simulink model "ddc_bpm_476_066"  (Simulink 7.8)
settings: Solver=ode45  StartTime=0.0  StopTime=2e-3  RelTol=1e-3
undefined symbols (not defined in the file): decim_factor_poly_35, dt_sim, frev_476, Fs_adc, n_ch, n_ovs, R_fofb, R_sec, R_sec_cfir, R_sec_pfir, xlipgetpartsetting
libraries: xbsIndex_r4 x1136, simulink x7
(part 2 of 10)

== system ddc_bpm_476_066/Ksum_tbt_mult2 ==
  In1 : Inport
  In2 : Inport  Port=2
  Cast_truncate1 : Subsystem
  Kx_tbt : xbsIndex_r4/Mult  precision=Full  arith_type="Signed  (2's comp)"  n_bits=16  bin_pt=14  quantization=Truncate  overflow=Wrap  en=off  latency=8  dbl_ovrd=off  use_behavioral_HDL=off  opt=Speed  use_embedded=off  optimum_pipeline=on  pipeline=on  use_rpm=on  placement_style=Triangular  block_type=mult
  Register : xbsIndex_r4/Register  init=0  rst=off  en=off  dbl_ovrd=off  block_type=register
  Out1 : Outport
  wires:
  Kx_tbt/1 -> Cast_truncate1/1(In1)
  In1/1 -> Kx_tbt/1
  Cast_truncate1/1(Out1) -> Register/1
  In2/1 -> Kx_tbt/2
  Register/1 -> Out1/1

== system ddc_bpm_476_066/Ksum_tbt_mult3 ==
  In1 : Inport
  In2 : Inport  Port=2
  Cast_truncate1 : Subsystem
  Kx_tbt : xbsIndex_r4/Mult  precision=Full  arith_type="Signed  (2's comp)"  n_bits=16  bin_pt=14  quantization=Truncate  overflow=Wrap  en=off  latency=8  dbl_ovrd=off  use_behavioral_HDL=off  opt=Speed  use_embedded=off  optimum_pipeline=on  pipeline=on  use_rpm=on  placement_style=Triangular  block_type=mult
  Register : xbsIndex_r4/Register  init=0  rst=off  en=off  dbl_ovrd=off  block_type=register
  Out1 : Outport
  wires:
  Kx_tbt/1 -> Cast_truncate1/1(In1)
  In1/1 -> Kx_tbt/1
  Cast_truncate1/1(Out1) -> Register/1
  In2/1 -> Kx_tbt/2
  Register/1 -> Out1/1

== system ddc_bpm_476_066/Kx_fofb_mult ==
  In1 : Inport
  In2 : Inport  Port=2
  Cast_truncate1 : Subsystem
  Kx_tbt : xbsIndex_r4/Mult  precision=Full  arith_type="Signed  (2's comp)"  n_bits=16  bin_pt=14  quantization=Truncate  overflow=Wrap  en=off  latency=8  dbl_ovrd=off  use_behavioral_HDL=off  opt=Speed  use_embedded=off  optimum_pipeline=on  pipeline=on  use_rpm=on  placement_style=Triangular  block_type=mult
  Register : xbsIndex_r4/Register  init=0  rst=off  en=off  dbl_ovrd=off  block_type=register
  Out1 : Outport
  wires:
  Kx_tbt/1 -> Cast_truncate1/1(In1)
  In1/1 -> Kx_tbt/1
  Cast_truncate1/1(Out1) -> Register/1
  In2/1 -> Kx_tbt/2
  Register/1 -> Out1/1

== system ddc_bpm_476_066/Kx_monit_mult ==
  In1 : Inport
  In2 : Inport  Port=2
  Cast_truncate1 : Subsystem
  Kx_tbt : xbsIndex_r4/Mult  precision=Full  arith_type="Signed  (2's comp)"  n_bits=16  bin_pt=14  quantization=Truncate  overflow=Wrap  en=off  latency=8  dbl_ovrd=off  use_behavioral_HDL=off  opt=Speed  use_embedded=off  optimum_pipeline=on  pipeline=on  use_rpm=on  placement_style=Triangular  block_type=mult
  Register : xbsIndex_r4/Register  init=0  rst=off  en=off  dbl_ovrd=off  block_type=register
  Out1 : Outport
  wires:
  Kx_tbt/1 -> Cast_truncate1/1(In1)
  In1/1 -> Kx_tbt/1
  Cast_truncate1/1(Out1) -> Register/1
  In2/1 -> Kx_tbt/2
  Register/1 -> Out1/1

== system ddc_bpm_476_066/Kx_monit_mult1 ==
  In1 : Inport
  In2 : Inport  Port=2
  Cast_truncate1 : Subsystem
  Kx_tbt : xbsIndex_r4/Mult  precision=Full  arith_type="Signed  (2's comp)"  n_bits=16  bin_pt=14  quantization=Truncate  overflow=Wrap  en=off  latency=8  dbl_ovrd=off  use_behavioral_HDL=off  opt=Speed  use_embedded=off  optimum_pipeline=on  pipeline=on  use_rpm=on  placement_style=Triangular  block_type=mult
  Register : xbsIndex_r4/Register  init=0  rst=off  en=off  dbl_ovrd=off  block_type=register
  Out1 : Outport
  wires:
  Kx_tbt/1 -> Cast_truncate1/1(In1)
  In1/1 -> Kx_tbt/1
  Cast_truncate1/1(Out1) -> Register/1
  In2/1 -> Kx_tbt/2
  Register/1 -> Out1/1

== system ddc_bpm_476_066/Kx_q_fofb_mult ==
  In1 : Inport
  In2 : Inport  Port=2
  Cast_truncate1 : Subsystem
  Kx_tbt : xbsIndex_r4/Mult  precision=Full  arith_type="Signed  (2's comp)"  n_bits=16  bin_pt=14  quantization=Truncate  overflow=Wrap  en=off  latency=8  dbl_ovrd=off  use_behavioral_HDL=off  opt=Speed  use_embedded=off  optimum_pipeline=on  pipeline=on  use_rpm=on  placement_style=Triangular  block_type=mult
  Register : xbsIndex_r4/Register  init=0  rst=off  en=off  dbl_ovrd=off  block_type=register
  Out1 : Outport
  wires:
  Kx_tbt/1 -> Cast_truncate1/1(In1)
  In1/1 -> Kx_tbt/1
  Cast_truncate1/1(Out1) -> Register/1
  In2/1 -> Kx_tbt/2
  Register/1 -> Out1/1

== system ddc_bpm_476_066/Kx_q_fofb_mult1 ==
  In1 : Inport
  In2 : Inport  Port=2
  Cast_truncate1 : Subsystem
  Kx_tbt : xbsIndex_r4/Mult  precision=Full  arith_type="Signed  (2's comp)"  n_bits=16  bin_pt=14  quantization=Truncate  overflow=Wrap  en=off  latency=8  dbl_ovrd=off  use_behavioral_HDL=off  opt=Speed  use_embedded=off  optimum_pipeline=on  pipeline=on  use_rpm=on  placement_style=Triangular  block_type=mult
  Register : xbsIndex_r4/Register  init=0  rst=off  en=off  dbl_ovrd=off  block_type=register
  Out1 : Outport
  wires:
  Kx_tbt/1 -> Cast_truncate1/1(In1)
  In1/1 -> Kx_tbt/1
  Cast_truncate1/1(Out1) -> Register/1
  In2/1 -> Kx_tbt/2
  Register/1 -> Out1/1

== system ddc_bpm_476_066/Kx_q_fofb_mult2 ==
  In1 : Inport
  In2 : Inport  Port=2
  Cast_truncate1 : Subsystem
  Kx_tbt : xbsIndex_r4/Mult  precision=Full  arith_type="Signed  (2's comp)"  n_bits=16  bin_pt=14  quantization=Truncate  overflow=Wrap  en=off  latency=8  dbl_ovrd=off  use_behavioral_HDL=off  opt=Speed  use_embedded=off  optimum_pipeline=on  pipeline=on  use_rpm=on  placement_style=Triangular  block_type=mult
  Register : xbsIndex_r4/Register  init=0  rst=off  en=off  dbl_ovrd=off  block_type=register
  Out1 : Outport
  wires:
  Kx_tbt/1 -> Cast_truncate1/1(In1)
  In1/1 -> Kx_tbt/1
  Cast_truncate1/1(Out1) -> Register/1
  In2/1 -> Kx_tbt/2
  Register/1 -> Out1/1

== system ddc_bpm_476_066/Kx_q_monit_mult ==
  In1 : Inport
  In2 : Inport  Port=2
  Cast_truncate1 : Subsystem
  Kx_tbt : xbsIndex_r4/Mult  precision=Full  arith_type="Signed  (2's comp)"  n_bits=16  bin_pt=14  quantization=Truncate  overflow=Wrap  en=off  latency=8  dbl_ovrd=off  use_behavioral_HDL=off  opt=Speed  use_embedded=off  optimum_pipeline=on  pipeline=on  use_rpm=on  placement_style=Triangular  block_type=mult
  Register : xbsIndex_r4/Register  init=0  rst=off  en=off  dbl_ovrd=off  block_type=register
  Out1 : Outport
  wires:
  Kx_tbt/1 -> Cast_truncate1/1(In1)
  In1/1 -> Kx_tbt/1
  Cast_truncate1/1(Out1) -> Register/1
  In2/1 -> Kx_tbt/2
  Register/1 -> Out1/1

== system ddc_bpm_476_066/Kx_q_monit_mult1 ==
  In1 : Inport
  In2 : Inport  Port=2
  Cast_truncate1 : Subsystem
  Kx_tbt : xbsIndex_r4/Mult  precision=Full  arith_type="Signed  (2's comp)"  n_bits=16  bin_pt=14  quantization=Truncate  overflow=Wrap  en=off  latency=8  dbl_ovrd=off  use_behavioral_HDL=off  opt=Speed  use_embedded=off  optimum_pipeline=on  pipeline=on  use_rpm=on  placement_style=Triangular  block_type=mult
  Register : xbsIndex_r4/Register  init=0  rst=off  en=off  dbl_ovrd=off  block_type=register
  Out1 : Outport
  wires:
  Kx_tbt/1 -> Cast_truncate1/1(In1)
  In1/1 -> Kx_tbt/1
  Cast_truncate1/1(Out1) -> Register/1
  In2/1 -> Kx_tbt/2
  Register/1 -> Out1/1

== system ddc_bpm_476_066/Kx_q_tbt_mult ==
  In1 : Inport
  In2 : Inport  Port=2
  Cast_truncate1 : Subsystem
  Kx_tbt : xbsIndex_r4/Mult  precision=Full  arith_type="Signed  (2's comp)"  n_bits=16  bin_pt=14  quantization=Truncate  overflow=Wrap  en=off  latency=8  dbl_ovrd=off  use_behavioral_HDL=off  opt=Speed  use_embedded=off  optimum_pipeline=on  pipeline=on  use_rpm=on  placement_style=Triangular  block_type=mult
  Register : xbsIndex_r4/Register  init=0  rst=off  en=off  dbl_ovrd=off  block_type=register
  Out1 : Outport
  wires:
  Kx_tbt/1 -> Cast_truncate1/1(In1)
  In1/1 -> Kx_tbt/1
  Cast_truncate1/1(Out1) -> Register/1
  In2/1 -> Kx_tbt/2
  Register/1 -> Out1/1

== system ddc_bpm_476_066/Kx_tbt_mult ==
  In1 : Inport
  In2 : Inport  Port=2
  Cast_truncate1 : Subsystem
  Kx_tbt : xbsIndex_r4/Mult  precision=Full  arith_type="Signed  (2's comp)"  n_bits=16  bin_pt=14  quantization=Truncate  overflow=Wrap  en=off  latency=8  dbl_ovrd=off  use_behavioral_HDL=off  opt=Speed  use_embedded=off  optimum_pipeline=on  pipeline=on  use_rpm=on  placement_style=Triangular  block_type=mult
  Register : xbsIndex_r4/Register  init=0  rst=off  en=off  dbl_ovrd=off  block_type=register
  Out1 : Outport
  wires:
  Kx_tbt/1 -> Cast_truncate1/1(In1)
  In1/1 -> Kx_tbt/1
  Cast_truncate1/1(Out1) -> Register/1
  In2/1 -> Kx_tbt/2
  Register/1 -> Out1/1

== system ddc_bpm_476_066/Ky_tbt_mult ==
  In1 : Inport
  In2 : Inport  Port=2
  Cast_truncate1 : Subsystem
  Ky_tbt : xbsIndex_r4/Mult  precision=Full  arith_type="Signed  (2's comp)"  n_bits=16  bin_pt=14  quantization=Truncate  overflow=Wrap  en=off  latency=8  dbl_ovrd=off  use_behavioral_HDL=off  opt=Speed  use_embedded=off  optimum_pipeline=on  pipeline=on  use_rpm=on  placement_style=Triangular  block_type=mult
  Register : xbsIndex_r4/Register  init=0  rst=off  en=off  dbl_ovrd=off  block_type=register
  Out1 : Outport
  wires:
  Ky_tbt/1 -> Cast_truncate1/1(In1)
  In1/1 -> Ky_tbt/1
  Cast_truncate1/1(Out1) -> Register/1
  In2/1 -> Ky_tbt/2
  Register/1 -> Out1/1

== system ddc_bpm_476_066/Ky_tbt_mult1 ==
  In1 : Inport
  In2 : Inport  Port=2
  Cast_truncate1 : Subsystem
  Kx_tbt : xbsIndex_r4/Mult  precision=Full  arith_type="Signed  (2's comp)"  n_bits=16  bin_pt=14  quantization=Truncate  overflow=Wrap  en=off  latency=8  dbl_ovrd=off  use_behavioral_HDL=off  opt=Speed  use_embedded=off  optimum_pipeline=on  pipeline=on  use_rpm=on  placement_style=Triangular  block_type=mult
  Register : xbsIndex_r4/Register  init=0  rst=off  en=off  dbl_ovrd=off  block_type=register
  Out1 : Outport
  wires:
  Kx_tbt/1 -> Cast_truncate1/1(In1)
  In1/1 -> Kx_tbt/1
  Cast_truncate1/1(Out1) -> Register/1
  In2/1 -> Kx_tbt/2
  Register/1 -> Out1/1

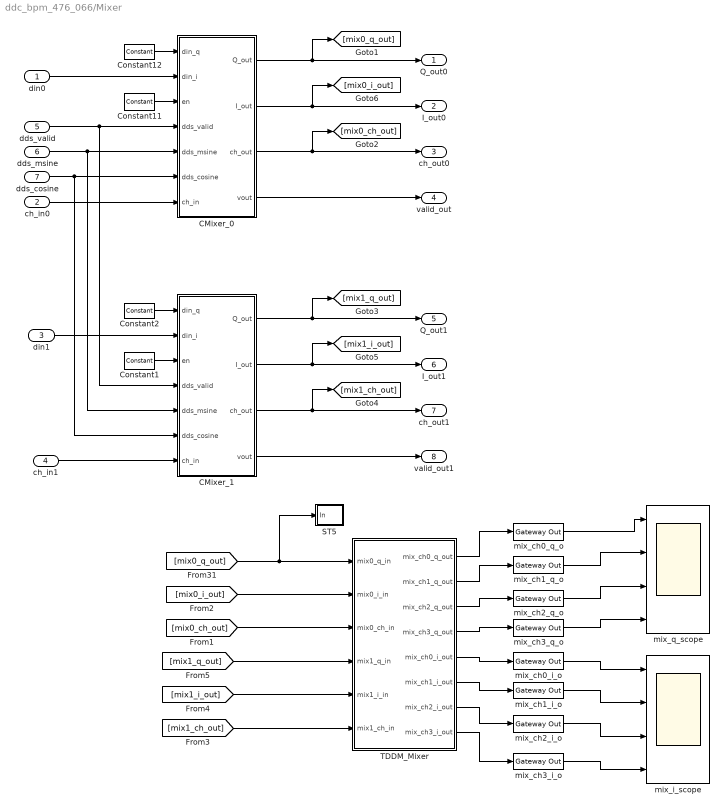
== system ddc_bpm_476_066/Mixer ==
  din0 : Inport
  ch_in0 : Inport  Port=2
  din1 : Inport  Port=3
  ch_in1 : Inport  Port=4
  dds_valid : Inport  Port=5
  dds_msine : Inport  Port=6
  dds_cosine : Inport  Port=7
  CMixer_0 : Subsystem
  CMixer_1 : Subsystem
  Constant1 : xbsIndex_r4/Constant  const=1  gui_display_data_type=Boolean  arith_type=Boolean  n_bits=24  bin_pt=22  preci_type=Single  exp_width=8  frac_width=24  explicit_period=on  period=dt_sim  equ=P=C  opselect=C  inp2=PCIN>>17  opr=+  inp1=P  carry=CIN  dbl_ovrd=off  block_type=constant
  Constant11 : xbsIndex_r4/Constant  const=1  gui_display_data_type=Boolean  arith_type=Boolean  n_bits=24  bin_pt=22  preci_type=Single  exp_width=8  frac_width=24  explicit_period=on  period=dt_sim  equ=P=C  opselect=C  inp2=PCIN>>17  opr=+  inp1=P  carry=CIN  dbl_ovrd=off  block_type=constant
  Constant12 : xbsIndex_r4/Constant  const=0  gui_display_data_type=Fixed-point  arith_type=Signed (2's comp)  n_bits=24  bin_pt=22  preci_type=Single  exp_width=8  frac_width=24  explicit_period=on  period=dt_sim  equ=P=C  opselect=C  inp2=PCIN>>17  opr=+  inp1=P  carry=CIN  dbl_ovrd=off  block_type=constant
  Constant2 : xbsIndex_r4/Constant  const=0  gui_display_data_type=Fixed-point  arith_type=Signed (2's comp)  n_bits=24  bin_pt=22  preci_type=Single  exp_width=8  frac_width=24  explicit_period=on  period=dt_sim  equ=P=C  opselect=C  inp2=PCIN>>17  opr=+  inp1=P  carry=CIN  dbl_ovrd=off  block_type=constant
  ST5 : Subsystem
  TDDM_Mixer : Subsystem
  mix_ch0_i_o : xbsIndex_r4/Gateway Out  inherit_from_input=on  hdl_port=on  timing_constraint=Data Rate  locs_specified=off  LOCs={}  UseAsDAC=off  DACChannel='1'  block_type=gatewayout
      settings: infoedit="Gateway out block.  Converts Xilinx fixed-point or floating-point type inputs into ouputs of type Simulink integer, single, double, or fixed point.<br><br>Hardware notes:  In hardware these blocks become top level output ports or are discarded, depending on how they are configured."
  mix_ch0_q_o : xbsIndex_r4/Gateway Out  inherit_from_input=on  hdl_port=on  timing_constraint=Data Rate  locs_specified=off  LOCs={}  UseAsDAC=off  DACChannel='1'  block_type=gatewayout
      settings: infoedit="Gateway out block.  Converts Xilinx fixed-point or floating-point type inputs into ouputs of type Simulink integer, single, double, or fixed point.<br><br>Hardware notes:  In hardware these blocks become top level output ports or are discarded, depending on how they are configured."
  mix_ch1_i_o : xbsIndex_r4/Gateway Out  inherit_from_input=on  hdl_port=on  timing_constraint=Data Rate  locs_specified=off  LOCs={}  UseAsDAC=off  DACChannel='1'  block_type=gatewayout
      settings: infoedit="Gateway out block.  Converts Xilinx fixed-point or floating-point type inputs into ouputs of type Simulink integer, single, double, or fixed point.<br><br>Hardware notes:  In hardware these blocks become top level output ports or are discarded, depending on how they are configured."
  mix_ch1_q_o : xbsIndex_r4/Gateway Out  inherit_from_input=on  hdl_port=on  timing_constraint=Data Rate  locs_specified=off  LOCs={}  UseAsDAC=off  DACChannel='1'  block_type=gatewayout
      settings: infoedit="Gateway out block.  Converts Xilinx fixed-point or floating-point type inputs into ouputs of type Simulink integer, single, double, or fixed point.<br><br>Hardware notes:  In hardware these blocks become top level output ports or are discarded, depending on how they are configured."
  mix_ch2_i_o : xbsIndex_r4/Gateway Out  inherit_from_input=on  hdl_port=on  timing_constraint=Data Rate  locs_specified=off  LOCs={}  UseAsDAC=off  DACChannel='1'  block_type=gatewayout
      settings: infoedit="Gateway out block.  Converts Xilinx fixed-point or floating-point type inputs into ouputs of type Simulink integer, single, double, or fixed point.<br><br>Hardware notes:  In hardware these blocks become top level output ports or are discarded, depending on how they are configured."
  mix_ch2_q_o : xbsIndex_r4/Gateway Out  inherit_from_input=on  hdl_port=on  timing_constraint=Data Rate  locs_specified=off  LOCs={}  UseAsDAC=off  DACChannel='1'  block_type=gatewayout
      settings: infoedit="Gateway out block.  Converts Xilinx fixed-point or floating-point type inputs into ouputs of type Simulink integer, single, double, or fixed point.<br><br>Hardware notes:  In hardware these blocks become top level output ports or are discarded, depending on how they are configured."
  mix_ch3_i_o : xbsIndex_r4/Gateway Out  inherit_from_input=on  hdl_port=on  timing_constraint=Data Rate  locs_specified=off  LOCs={}  UseAsDAC=off  DACChannel='1'  block_type=gatewayout
      settings: infoedit="Gateway out block.  Converts Xilinx fixed-point or floating-point type inputs into ouputs of type Simulink integer, single, double, or fixed point.<br><br>Hardware notes:  In hardware these blocks become top level output ports or are discarded, depending on how they are configured."
  mix_ch3_q_o : xbsIndex_r4/Gateway Out  inherit_from_input=on  hdl_port=on  timing_constraint=Data Rate  locs_specified=off  LOCs={}  UseAsDAC=off  DACChannel='1'  block_type=gatewayout
      settings: infoedit="Gateway out block.  Converts Xilinx fixed-point or floating-point type inputs into ouputs of type Simulink integer, single, double, or fixed point.<br><br>Hardware notes:  In hardware these blocks become top level output ports or are discarded, depending on how they are configured."
  mix_i_scope : Scope  NumInputPorts=4
      settings: TimeRange=0.00011214  YMin=-0.1~-1.5~-0.002~-1.5  YMax=1~1.5~0.00075~1.5  SaveName=ScopeData14  MaxDataPoints=1000000  SampleInput=on
  mix_q_scope : Scope  NumInputPorts=4
      settings: TimeRange=0.00011214  YMin=-0.1~-1.5~-0.002~-1.5  YMax=1~1.5~0.00075~1.5  SaveName=ScopeData13  MaxDataPoints=1000000  SampleInput=on
  Q_out0 : Outport
  I_out0 : Outport  Port=2
  ch_out0 : Outport  Port=3
  valid_out : Outport  Port=4
  Q_out1 : Outport  Port=5
  I_out1 : Outport  Port=6
  ch_out1 : Outport  Port=7
  valid_out1 : Outport  Port=8
  wires:
  Constant12/1 -> CMixer_0/1(din_q)
  Constant11/1 -> CMixer_0/3(en)
  CMixer_0/1(Q_out) -> Q_out0/1, [mix0_q_out]
  din0/1 -> CMixer_0/2(din_i)
  CMixer_0/2(I_out) -> I_out0/1, [mix0_i_out]
  dds_valid/1 -> CMixer_0/4(dds_valid), CMixer_1/4(dds_valid)
  dds_cosine/1 -> CMixer_0/6(dds_cosine), CMixer_1/6(dds_cosine)
  CMixer_0/3(ch_out) -> ch_out0/1, [mix0_ch_out]
  dds_msine/1 -> CMixer_0/5(dds_msine), CMixer_1/5(dds_msine)
  CMixer_0/4(vout) -> valid_out/1
  ch_in0/1 -> CMixer_0/7(ch_in)
  [mix0_q_out] -> TDDM_Mixer/1(mix0_q_in), ST5/1(In)
  [mix0_ch_out] -> TDDM_Mixer/3(mix0_ch_in)
  [mix0_i_out] -> TDDM_Mixer/2(mix0_i_in)
  TDDM_Mixer/1(mix_ch0_q_out) -> mix_ch0_q_o/1
  TDDM_Mixer/2(mix_ch1_q_out) -> mix_ch1_q_o/1
  TDDM_Mixer/3(mix_ch2_q_out) -> mix_ch2_q_o/1
  TDDM_Mixer/4(mix_ch3_q_out) -> mix_ch3_q_o/1
  TDDM_Mixer/5(mix_ch0_i_out) -> mix_ch0_i_o/1
  TDDM_Mixer/6(mix_ch1_i_out) -> mix_ch1_i_o/1
  TDDM_Mixer/7(mix_ch2_i_out) -> mix_ch2_i_o/1
  TDDM_Mixer/8(mix_ch3_i_out) -> mix_ch3_i_o/1
  mix_ch0_i_o/1 -> mix_i_scope/1
  mix_ch1_i_o/1 -> mix_i_scope/2
  mix_ch2_i_o/1 -> mix_i_scope/3
  mix_ch3_i_o/1 -> mix_i_scope/4
  mix_ch3_q_o/1 -> mix_q_scope/4
  mix_ch2_q_o/1 -> mix_q_scope/3
  mix_ch1_q_o/1 -> mix_q_scope/2
  mix_ch0_q_o/1 -> mix_q_scope/1
  Constant2/1 -> CMixer_1/1(din_q)
  Constant1/1 -> CMixer_1/3(en)
  CMixer_1/1(Q_out) -> Q_out1/1, [mix1_q_out]
  din1/1 -> CMixer_1/2(din_i)
  CMixer_1/2(I_out) -> I_out1/1, [mix1_i_out]
  CMixer_1/3(ch_out) -> ch_out1/1, [mix1_ch_out]
  CMixer_1/4(vout) -> valid_out1/1
  ch_in1/1 -> CMixer_1/7(ch_in)
  [mix1_q_out] -> TDDM_Mixer/4(mix1_q_in)
  [mix1_i_out] -> TDDM_Mixer/5(mix1_i_in)
  [mix1_ch_out] -> TDDM_Mixer/6(mix1_ch_in)

== system ddc_bpm_476_066/Monit_amp ==
  din : Inport
  ch_in : Inport  Port=2
  Monit_amp_c : Subsystem
  TDDM_monit_amp_out : Subsystem
  Terminator5 : Terminator
  amp_out0 : Outport
  amp_out1 : Outport  Port=2
  amp_out2 : Outport  Port=3
  amp_out3 : Outport  Port=4
  wires:
  Monit_amp_c/1(amp_out) -> TDDM_monit_amp_out/1(monit_amp_din)
  Monit_amp_c/2(ch_out) -> TDDM_monit_amp_out/2(monit_amp_ch_in)
  Monit_amp_c/3(valid_out) -> Terminator5/1
  TDDM_monit_amp_out/1(monit_amp_data0_out) -> amp_out0/1
  din/1 -> Monit_amp_c/1(din)
  TDDM_monit_amp_out/2(monit_amp_data1_out) -> amp_out1/1
  TDDM_monit_amp_out/3(monit_amp_data2_out) -> amp_out2/1
  ch_in/1 -> Monit_amp_c/2(ch_in)
  TDDM_monit_amp_out/4(monit_amp_data3_out) -> amp_out3/1

== system ddc_bpm_476_066/ST1 ==
  In : Inport
  Display : Display
  Sample Time : xbsIndex_r4/Sample Time  block_type=sampletime
      settings: infoedit="The Sample Time block reports the normalized sample period of its input.  A signal's normalized sample period is not equivalent to its Simulink absolute sample period.<br><br>Hardware notes: This block is implemented as a constant in hardware."
  out : xbsIndex_r4/Gateway Out  inherit_from_input=on  hdl_port=off  timing_constraint=Data Rate  locs_specified=off  LOCs={}  UseAsDAC=off  DACChannel='1'  block_type=gatewayout
      settings: infoedit="Gateway out block.  Converts Xilinx fixed-point or floating-point type inputs into ouputs of type Simulink integer, single, double, or fixed point.<br><br>Hardware notes:  In hardware these blocks become top level output ports or are discarded, depending on how they are configured."
  wires:
  out/1 -> Display/1
  Sample Time/1 -> out/1
  In/1 -> Sample Time/1

== system ddc_bpm_476_066/ST10 ==
  In : Inport
  Display : Display
  Sample Time : xbsIndex_r4/Sample Time  block_type=sampletime
      settings: infoedit="The Sample Time block reports the normalized sample period of its input.  A signal's normalized sample period is not equivalent to its Simulink absolute sample period.<br><br>Hardware notes: This block is implemented as a constant in hardware."
  out : xbsIndex_r4/Gateway Out  inherit_from_input=on  hdl_port=off  timing_constraint=Data Rate  locs_specified=off  LOCs={}  UseAsDAC=off  DACChannel='1'  block_type=gatewayout
      settings: infoedit="Gateway out block.  Converts Xilinx fixed-point or floating-point type inputs into ouputs of type Simulink integer, single, double, or fixed point.<br><br>Hardware notes:  In hardware these blocks become top level output ports or are discarded, depending on how they are configured."
  wires:
  out/1 -> Display/1
  Sample Time/1 -> out/1
  In/1 -> Sample Time/1

== system ddc_bpm_476_066/ST2 ==
  In : Inport
  Display : Display
  Sample Time : xbsIndex_r4/Sample Time  block_type=sampletime
      settings: infoedit="The Sample Time block reports the normalized sample period of its input.  A signal's normalized sample period is not equivalent to its Simulink absolute sample period.<br><br>Hardware notes: This block is implemented as a constant in hardware."
  out : xbsIndex_r4/Gateway Out  inherit_from_input=on  hdl_port=off  timing_constraint=Data Rate  locs_specified=off  LOCs={}  UseAsDAC=off  DACChannel='1'  block_type=gatewayout
      settings: infoedit="Gateway out block.  Converts Xilinx fixed-point or floating-point type inputs into ouputs of type Simulink integer, single, double, or fixed point.<br><br>Hardware notes:  In hardware these blocks become top level output ports or are discarded, depending on how they are configured."
  wires:
  out/1 -> Display/1
  Sample Time/1 -> out/1
  In/1 -> Sample Time/1

== system ddc_bpm_476_066/ST3 ==
  In : Inport
  Display : Display
  Sample Time : xbsIndex_r4/Sample Time  block_type=sampletime
      settings: infoedit="The Sample Time block reports the normalized sample period of its input.  A signal's normalized sample period is not equivalent to its Simulink absolute sample period.<br><br>Hardware notes: This block is implemented as a constant in hardware."
  out : xbsIndex_r4/Gateway Out  inherit_from_input=on  hdl_port=off  timing_constraint=Data Rate  locs_specified=off  LOCs={}  UseAsDAC=off  DACChannel='1'  block_type=gatewayout
      settings: infoedit="Gateway out block.  Converts Xilinx fixed-point or floating-point type inputs into ouputs of type Simulink integer, single, double, or fixed point.<br><br>Hardware notes:  In hardware these blocks become top level output ports or are discarded, depending on how they are configured."
  wires:
  out/1 -> Display/1
  Sample Time/1 -> out/1
  In/1 -> Sample Time/1

== system ddc_bpm_476_066/ST4 ==
  In : Inport
  Display : Display
  Sample Time : xbsIndex_r4/Sample Time  block_type=sampletime
      settings: infoedit="The Sample Time block reports the normalized sample period of its input.  A signal's normalized sample period is not equivalent to its Simulink absolute sample period.<br><br>Hardware notes: This block is implemented as a constant in hardware."
  out : xbsIndex_r4/Gateway Out  inherit_from_input=on  hdl_port=off  timing_constraint=Data Rate  locs_specified=off  LOCs={}  UseAsDAC=off  DACChannel='1'  block_type=gatewayout
      settings: infoedit="Gateway out block.  Converts Xilinx fixed-point or floating-point type inputs into ouputs of type Simulink integer, single, double, or fixed point.<br><br>Hardware notes:  In hardware these blocks become top level output ports or are discarded, depending on how they are configured."
  wires:
  out/1 -> Display/1
  Sample Time/1 -> out/1
  In/1 -> Sample Time/1

== system ddc_bpm_476_066/ST5 ==
  In : Inport
  Display : Display
  Sample Time : xbsIndex_r4/Sample Time  block_type=sampletime
      settings: infoedit="The Sample Time block reports the normalized sample period of its input.  A signal's normalized sample period is not equivalent to its Simulink absolute sample period.<br><br>Hardware notes: This block is implemented as a constant in hardware."
  out : xbsIndex_r4/Gateway Out  inherit_from_input=on  hdl_port=off  timing_constraint=Data Rate  locs_specified=off  LOCs={}  UseAsDAC=off  DACChannel='1'  block_type=gatewayout
      settings: infoedit="Gateway out block.  Converts Xilinx fixed-point or floating-point type inputs into ouputs of type Simulink integer, single, double, or fixed point.<br><br>Hardware notes:  In hardware these blocks become top level output ports or are discarded, depending on how they are configured."
  wires:
  out/1 -> Display/1
  Sample Time/1 -> out/1
  In/1 -> Sample Time/1

== system ddc_bpm_476_066/ST6 ==
  In : Inport
  Display : Display
  Sample Time : xbsIndex_r4/Sample Time  block_type=sampletime
      settings: infoedit="The Sample Time block reports the normalized sample period of its input.  A signal's normalized sample period is not equivalent to its Simulink absolute sample period.<br><br>Hardware notes: This block is implemented as a constant in hardware."
  out : xbsIndex_r4/Gateway Out  inherit_from_input=on  hdl_port=off  timing_constraint=Data Rate  locs_specified=off  LOCs={}  UseAsDAC=off  DACChannel='1'  block_type=gatewayout
      settings: infoedit="Gateway out block.  Converts Xilinx fixed-point or floating-point type inputs into ouputs of type Simulink integer, single, double, or fixed point.<br><br>Hardware notes:  In hardware these blocks become top level output ports or are discarded, depending on how they are configured."
  wires:
  out/1 -> Display/1
  Sample Time/1 -> out/1
  In/1 -> Sample Time/1

== system ddc_bpm_476_066/ST7 ==
  In : Inport
  Display : Display
  Sample Time : xbsIndex_r4/Sample Time  block_type=sampletime
      settings: infoedit="The Sample Time block reports the normalized sample period of its input.  A signal's normalized sample period is not equivalent to its Simulink absolute sample period.<br><br>Hardware notes: This block is implemented as a constant in hardware."
  out : xbsIndex_r4/Gateway Out  inherit_from_input=on  hdl_port=off  timing_constraint=Data Rate  locs_specified=off  LOCs={}  UseAsDAC=off  DACChannel='1'  block_type=gatewayout
      settings: infoedit="Gateway out block.  Converts Xilinx fixed-point or floating-point type inputs into ouputs of type Simulink integer, single, double, or fixed point.<br><br>Hardware notes:  In hardware these blocks become top level output ports or are discarded, depending on how they are configured."
  wires:
  out/1 -> Display/1
  Sample Time/1 -> out/1
  In/1 -> Sample Time/1

== system ddc_bpm_476_066/ST8 ==
  In : Inport
  Display : Display
  Sample Time : xbsIndex_r4/Sample Time  block_type=sampletime
      settings: infoedit="The Sample Time block reports the normalized sample period of its input.  A signal's normalized sample period is not equivalent to its Simulink absolute sample period.<br><br>Hardware notes: This block is implemented as a constant in hardware."
  X_monit1 : xbsIndex_r4/Gateway Out  inherit_from_input=on  hdl_port=off  timing_constraint=Data Rate  locs_specified=off  LOCs={}  UseAsDAC=off  DACChannel='1'  block_type=gatewayout
      settings: infoedit="Gateway out block.  Converts Xilinx fixed-point or floating-point type inputs into ouputs of type Simulink integer, single, double, or fixed point.<br><br>Hardware notes:  In hardware these blocks become top level output ports or are discarded, depending on how they are configured."
  wires:
  X_monit1/1 -> Display/1
  Sample Time/1 -> X_monit1/1
  In/1 -> Sample Time/1

== system ddc_bpm_476_066/ST9 ==
  In : Inport
  Display : Display
  Sample Time : xbsIndex_r4/Sample Time  block_type=sampletime
      settings: infoedit="The Sample Time block reports the normalized sample period of its input.  A signal's normalized sample period is not equivalent to its Simulink absolute sample period.<br><br>Hardware notes: This block is implemented as a constant in hardware."
  out : xbsIndex_r4/Gateway Out  inherit_from_input=on  hdl_port=off  timing_constraint=Data Rate  locs_specified=off  LOCs={}  UseAsDAC=off  DACChannel='1'  block_type=gatewayout
      settings: infoedit="Gateway out block.  Converts Xilinx fixed-point or floating-point type inputs into ouputs of type Simulink integer, single, double, or fixed point.<br><br>Hardware notes:  In hardware these blocks become top level output ports or are discarded, depending on how they are configured."
  wires:
  out/1 -> Display/1
  Sample Time/1 -> out/1
  In/1 -> Sample Time/1

== system ddc_bpm_476_066/TBT_amp ==
  Q_in0 : Inport
  I_in0 : Inport  Port=2
  ch_in0 : Inport  Port=3
  Q_in1 : Inport  Port=4
  I_in1 : Inport  Port=5
  ch_in1 : Inport  Port=6
  ST5 : Subsystem
  TBT_amp0 : Subsystem
  TBT_amp1 : Subsystem
  TDDM_tbt_amp_4ch : Subsystem
  Terminator{,1,3..4} (4 alike) : Terminator
  amp_out0 : Outport
  amp_out1 : Outport  Port=2
  amp_out2 : Outport  Port=3
  amp_out3 : Outport  Port=4
  wires:
  Q_in0/1 -> TBT_amp0/1(Q_in)
  I_in0/1 -> TBT_amp0/2(I_in)
  ch_in0/1 -> TBT_amp0/3(ch_in)
  Q_in1/1 -> TBT_amp1/1(Q_in)
  I_in1/1 -> TBT_amp1/2(I_in)
  ch_in1/1 -> TBT_amp1/3(ch_in)
  TBT_amp0/2(phase_out) -> Terminator/1
  TBT_amp0/3(valid_out) -> Terminator1/1
  TBT_amp1/2(phase_out) -> Terminator3/1
  TBT_amp1/3(valid_out) -> Terminator4/1
  TBT_amp0/1(amp_out) -> TDDM_tbt_amp_4ch/1(amp_in0), ST5/1(In)
  TBT_amp0/4(ch_out) -> TDDM_tbt_amp_4ch/2(ch_in0)
  TBT_amp1/1(amp_out) -> TDDM_tbt_amp_4ch/3(amp_in1)
  TBT_amp1/4(ch_out) -> TDDM_tbt_amp_4ch/4(ch_in1)
  TDDM_tbt_amp_4ch/1(amp_out0) -> amp_out0/1
  TDDM_tbt_amp_4ch/2(amp_out1) -> amp_out1/1
  TDDM_tbt_amp_4ch/3(amp_out2) -> amp_out2/1
  TDDM_tbt_amp_4ch/4(amp_out3) -> amp_out3/1

== system ddc_bpm_476_066/TDM_mix ==
  din_ch0 : Inport
  din_ch1 : Inport  Port=2
  din_ch2 : Inport  Port=3
  din_ch3 : Inport  Port=4
  Constant10 : xbsIndex_r4/Constant  const=0  gui_display_data_type=Boolean  arith_type=Boolean  n_bits=16  bin_pt=14  preci_type=Single  exp_width=8  frac_width=24  explicit_period=on  period=1/Fs_adc/n_ovs  equ=P=C  opselect=C  inp2=PCIN>>17  opr=+  inp1=P  carry=CIN  dbl_ovrd=off  block_type=constant
  Constant11 : xbsIndex_r4/Constant  const=0  gui_display_data_type=Boolean  arith_type=Boolean  n_bits=16  bin_pt=14  preci_type=Single  exp_width=8  frac_width=24  explicit_period=on  period=1/Fs_adc/n_ovs  equ=P=C  opselect=C  inp2=PCIN>>17  opr=+  inp1=P  carry=CIN  dbl_ovrd=off  block_type=constant
  ST1 : Subsystem
  ST2 : Subsystem
  ST3 : Subsystem
  ST4 : Subsystem
  ST5 : Subsystem
  ST6 : Subsystem
  TDM_mix_ch0_1 : Subsystem
  TDM_mix_ch1_2 : Subsystem
  dout0 : Outport
  ch_out0 : Outport  Port=2
  dout1 : Outport  Port=3
  ch_out1 : Outport  Port=4
  wires:
  Constant10/1 -> TDM_mix_ch0_1/1(rst), ST3/1(In)
  Constant11/1 -> TDM_mix_ch1_2/1(rst), ST5/1(In)
  TDM_mix_ch0_1/1(dout) -> dout0/1, ST1/1(In)
  din_ch0/1 -> TDM_mix_ch0_1/2(din_ch0)
  TDM_mix_ch0_1/2(ch_out) -> ch_out0/1
  din_ch1/1 -> TDM_mix_ch0_1/3(din_ch1), ST2/1(In)
  TDM_mix_ch1_2/1(dout) -> dout1/1, ST4/1(In)
  din_ch2/1 -> TDM_mix_ch1_2/2(din_ch0)
  TDM_mix_ch1_2/2(ch_out) -> ch_out1/1
  din_ch3/1 -> TDM_mix_ch1_2/3(din_ch1), ST6/1(In)

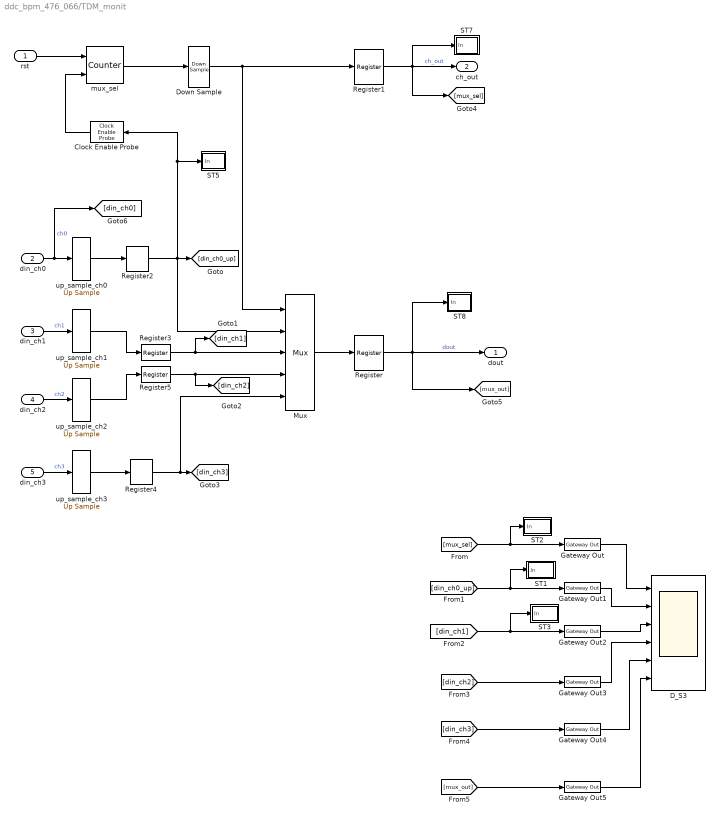
== system ddc_bpm_476_066/TDM_monit ==
  rst : Inport
  din_ch0 : Inport  Port=2
  din_ch1 : Inport  Port=3
  din_ch2 : Inport  Port=4
  din_ch3 : Inport  Port=5
  Clock Enable Probe : xbsIndex_r4/Clock Enable Probe  inherit_constraints=on  block_type=ceprobe
      settings: infoedit="Clock enable extractor.  Produces a Boolean output that mirrors the hardware clock enable associated with the input sample rate.<br><br>Hardware notes: in hardware this block costs nothing."
  D_S3 : Scope  NumInputPorts=6
      settings: TimeRange=0.0004  YMin=-1~-1.5~10~-1.5~-5~-5  YMax=1~1.5~100~1.5~5~5  MaxDataPoints=1000000  SampleInput=on
  Down Sample : xbsIndex_r4/Down Sample  sample_ratio=R_fofb*n_ovs/n_ch  sample_phase="Last Value of Frame  (most efficient)"  en=off  latency=1  dbl_ovrd=off  block_type=dsamp
  Gateway Out{,1..5} (6 alike) : xbsIndex_r4/Gateway Out  inherit_from_input=on  hdl_port=off  timing_constraint=None  locs_specified=off  LOCs={}  UseAsDAC=off  DACChannel='1'  block_type=gatewayout
      settings: infoedit="Gateway out block.  Converts Xilinx fixed-point or floating-point type inputs into ouputs of type Simulink integer, single, double, or fixed point.<br><br>Hardware notes:  In hardware these blocks become top level output ports or are discarded, depending on how they are configured."
  Mux : xbsIndex_r4/Mux  inputs=4  en=off  latency=0  precision=Full  arith_type=Unsigned  n_bits=16  bin_pt=14  quantization=Truncate  overflow=Wrap  dbl_ovrd=off  block_type=mux
  Register{,1..5} (6 alike) : xbsIndex_r4/Register  init=0  rst=off  en=off  dbl_ovrd=off  block_type=register
  ST1 : Subsystem
  ST2 : Subsystem
  ST3 : Subsystem
  ST5 : Subsystem
  ST7 : Subsystem
  ST8 : Subsystem
  mux_sel : xbsIndex_r4/Counter  cnt_type=Free Running  cnt_to=Inf  operation=Up  start_count=0  cnt_by_val=1  arith_type=Unsigned  n_bits=2  bin_pt=0  load_pin=off  rst=on  en=on  explicit_period=off  period=1/Fs_adc/4*1112  dbl_ovrd=off  use_behavioral_HDL=off  implementation=Fabric  block_type=counter
  up_sample_ch{0..3} (4 alike) : xbsIndex_r4/Up Sample  sample_ratio=n_ch  copy_samples=on  en=off  latency=0  dbl_ovrd=off  block_type=usamp
  dout : Outport
  ch_out : Outport  Port=2
  wires:
  Mux/1 -> Register/1
  mux_sel/1 -> Down Sample/1
  up_sample_ch3/1 -> Register4/1
  up_sample_ch2/1 -> Register5/1
  up_sample_ch1/1 -> Register3/1
  up_sample_ch0/1 -> Register2/1
  din_ch0/1 -> [din_ch0], up_sample_ch0/1  "ch0"
  din_ch1/1 -> up_sample_ch1/1  "ch1"
  Register/1 -> dout/1, [mux_out], ST8/1(In)  "dout"
  din_ch2/1 -> up_sample_ch2/1  "ch2"
  din_ch3/1 -> up_sample_ch3/1  "ch3"
  Register1/1 -> ch_out/1, [mux_sel], ST7/1(In)  "ch_out"
  Gateway Out/1 -> D_S3/1
  Gateway Out1/1 -> D_S3/2
  Gateway Out4/1 -> D_S3/5
  Gateway Out3/1 -> D_S3/4
  Gateway Out2/1 -> D_S3/3
  [mux_sel] -> Gateway Out/1, ST2/1(In)
  [din_ch0_up] -> Gateway Out1/1, ST1/1(In)
  [din_ch1] -> Gateway Out2/1, ST3/1(In)
  [din_ch3] -> Gateway Out4/1
  [din_ch2] -> Gateway Out3/1
  [mux_out] -> Gateway Out5/1
  Gateway Out5/1 -> D_S3/6
  Register2/1 -> Mux/2, [din_ch0_up], Clock Enable Probe/1, ST5/1(In)
  Register3/1 -> Mux/3, [din_ch1]
  Register4/1 -> Mux/5, [din_ch3]
  Register5/1 -> Mux/4, [din_ch2]
  Clock Enable Probe/1 -> mux_sel/2
  rst/1 -> mux_sel/1
  Down Sample/1 -> Register1/1, Mux/1

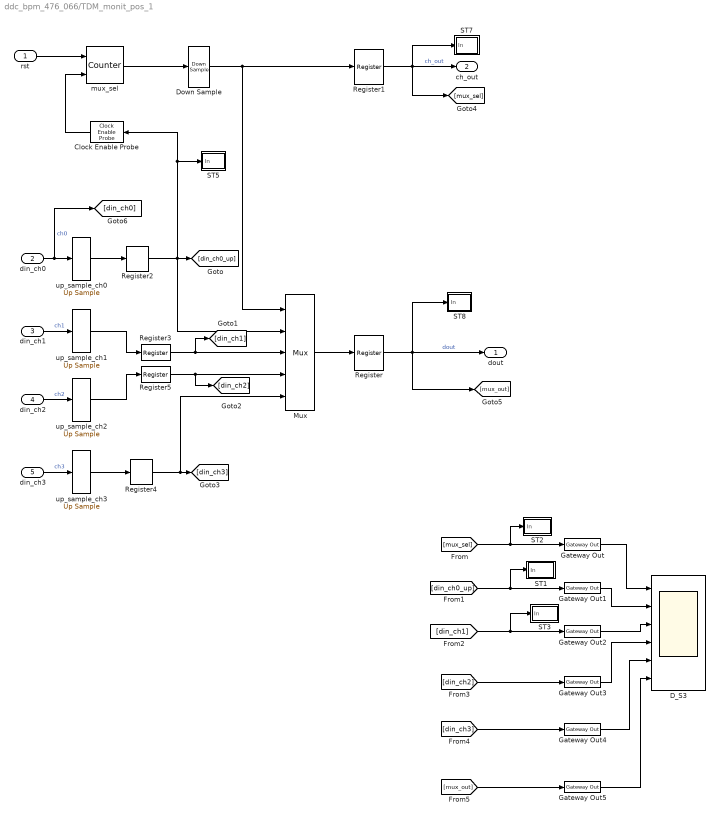
== system ddc_bpm_476_066/TDM_monit_pos_1 ==
  rst : Inport
  din_ch0 : Inport  Port=2
  din_ch1 : Inport  Port=3
  din_ch2 : Inport  Port=4
  din_ch3 : Inport  Port=5
  Clock Enable Probe : xbsIndex_r4/Clock Enable Probe  inherit_constraints=on  block_type=ceprobe
      settings: infoedit="Clock enable extractor.  Produces a Boolean output that mirrors the hardware clock enable associated with the input sample rate.<br><br>Hardware notes: in hardware this block costs nothing."
  D_S3 : Scope  NumInputPorts=6
      settings: TimeRange=0.0004  YMin=-1~-1.5~10~-1.5~-5~-5  YMax=1~1.5~100~1.5~5~5  MaxDataPoints=1000000  SampleInput=on
  Down Sample : xbsIndex_r4/Down Sample  sample_ratio=R_fofb*R_sec*R_sec_cfir*R_sec_pfir*n_ovs/n_ch  sample_phase="Last Value of Frame  (most efficient)"  en=off  latency=1  dbl_ovrd=off  block_type=dsamp
  Gateway Out{,1..5} (6 alike) : xbsIndex_r4/Gateway Out  inherit_from_input=on  hdl_port=off  timing_constraint=None  locs_specified=off  LOCs={}  UseAsDAC=off  DACChannel='1'  block_type=gatewayout
      settings: infoedit="Gateway out block.  Converts Xilinx fixed-point or floating-point type inputs into ouputs of type Simulink integer, single, double, or fixed point.<br><br>Hardware notes:  In hardware these blocks become top level output ports or are discarded, depending on how they are configured."
  Mux : xbsIndex_r4/Mux  inputs=4  en=off  latency=0  precision=Full  arith_type=Unsigned  n_bits=16  bin_pt=14  quantization=Truncate  overflow=Wrap  dbl_ovrd=off  block_type=mux
  Register{,1..5} (6 alike) : xbsIndex_r4/Register  init=0  rst=off  en=off  dbl_ovrd=off  block_type=register
  ST1 : Subsystem
  ST2 : Subsystem
  ST3 : Subsystem
  ST5 : Subsystem
  ST7 : Subsystem
  ST8 : Subsystem
  mux_sel : xbsIndex_r4/Counter  cnt_type=Free Running  cnt_to=Inf  operation=Up  start_count=0  cnt_by_val=1  arith_type=Unsigned  n_bits=2  bin_pt=0  load_pin=off  rst=on  en=on  explicit_period=off  period=1/Fs_adc/4*1112  dbl_ovrd=off  use_behavioral_HDL=off  implementation=Fabric  block_type=counter
  up_sample_ch{0..3} (4 alike) : xbsIndex_r4/Up Sample  sample_ratio=n_ch  copy_samples=on  en=off  latency=0  dbl_ovrd=off  block_type=usamp
  dout : Outport
  ch_out : Outport  Port=2
  wires:
  Mux/1 -> Register/1
  mux_sel/1 -> Down Sample/1
  up_sample_ch3/1 -> Register4/1
  up_sample_ch2/1 -> Register5/1
  up_sample_ch1/1 -> Register3/1
  up_sample_ch0/1 -> Register2/1
  din_ch0/1 -> [din_ch0], up_sample_ch0/1  "ch0"
  din_ch1/1 -> up_sample_ch1/1  "ch1"
  Register/1 -> dout/1, [mux_out], ST8/1(In)  "dout"
  din_ch2/1 -> up_sample_ch2/1  "ch2"
  din_ch3/1 -> up_sample_ch3/1  "ch3"
  Register1/1 -> ch_out/1, [mux_sel], ST7/1(In)  "ch_out"
  Gateway Out/1 -> D_S3/1
  Gateway Out1/1 -> D_S3/2
  Gateway Out4/1 -> D_S3/5
  Gateway Out3/1 -> D_S3/4
  Gateway Out2/1 -> D_S3/3
  [mux_sel] -> Gateway Out/1, ST2/1(In)
  [din_ch0_up] -> Gateway Out1/1, ST1/1(In)
  [din_ch1] -> Gateway Out2/1, ST3/1(In)
  [din_ch3] -> Gateway Out4/1
  [din_ch2] -> Gateway Out3/1
  [mux_out] -> Gateway Out5/1
  Gateway Out5/1 -> D_S3/6
  Register2/1 -> Mux/2, [din_ch0_up], Clock Enable Probe/1, ST5/1(In)
  Register3/1 -> Mux/3, [din_ch1]
  Register4/1 -> Mux/5, [din_ch3]
  Register5/1 -> Mux/4, [din_ch2]
  Clock Enable Probe/1 -> mux_sel/2
  rst/1 -> mux_sel/1
  Down Sample/1 -> Register1/1, Mux/1

== system ddc_bpm_476_066/debug_analysis ==
  Constant{,1..3} (4 alike) : Constant  Value=0
  D_S2 : Scope  NumInputPorts=2
      settings: TimeRange=0.0004  YMin=1~1  YMax=1~1  SaveName=ScopeData8  MaxDataPoints=1000000  SampleInput=on
  D_S3 : Scope  NumInputPorts=4
      settings: TimeRange=0.0004  YMin=-1~-1.5~10~-1.5  YMax=1~1.5~100~1.5  SaveName=ScopeData9  MaxDataPoints=1000000  SampleInput=on
  D_S4 : Scope  NumInputPorts=4
      settings: TimeRange=0.0004  YMin=0.95~0~10~-1.5  YMax=1.05~60~100~1.5  SaveName=ScopeData10  MaxDataPoints=1000000  SampleInput=on
  q_tbt_o3 : xbsIndex_r4/Gateway Out  inherit_from_input=on  hdl_port=off  timing_constraint=None  locs_specified=off  LOCs={}  UseAsDAC=off  DACChannel='1'  block_type=gatewayout
      settings: infoedit="Gateway out block.  Converts Xilinx fixed-point or floating-point type inputs into ouputs of type Simulink integer, single, double, or fixed point.<br><br>Hardware notes:  In hardware these blocks become top level output ports or are discarded, depending on how they are configured."
  sum_tbt_o3 : xbsIndex_r4/Gateway Out  inherit_from_input=on  hdl_port=off  timing_constraint=None  locs_specified=off  LOCs={}  UseAsDAC=off  DACChannel='1'  block_type=gatewayout
      settings: infoedit="Gateway out block.  Converts Xilinx fixed-point or floating-point type inputs into ouputs of type Simulink integer, single, double, or fixed point.<br><br>Hardware notes:  In hardware these blocks become top level output ports or are discarded, depending on how they are configured."
  x_tbt_o3 : xbsIndex_r4/Gateway Out  inherit_from_input=on  hdl_port=off  timing_constraint=None  locs_specified=off  LOCs={}  UseAsDAC=off  DACChannel='1'  block_type=gatewayout
      settings: infoedit="Gateway out block.  Converts Xilinx fixed-point or floating-point type inputs into ouputs of type Simulink integer, single, double, or fixed point.<br><br>Hardware notes:  In hardware these blocks become top level output ports or are discarded, depending on how they are configured."
  x_tbt_o4 : xbsIndex_r4/Gateway Out  inherit_from_input=on  hdl_port=off  timing_constraint=None  locs_specified=off  LOCs={}  UseAsDAC=off  DACChannel='1'  block_type=gatewayout
      settings: infoedit="Gateway out block.  Converts Xilinx fixed-point or floating-point type inputs into ouputs of type Simulink integer, single, double, or fixed point.<br><br>Hardware notes:  In hardware these blocks become top level output ports or are discarded, depending on how they are configured."
  y_tbt_o4 : xbsIndex_r4/Gateway Out  inherit_from_input=on  hdl_port=off  timing_constraint=None  locs_specified=off  LOCs={}  UseAsDAC=off  DACChannel='1'  block_type=gatewayout
      settings: infoedit="Gateway out block.  Converts Xilinx fixed-point or floating-point type inputs into ouputs of type Simulink integer, single, double, or fixed point.<br><br>Hardware notes:  In hardware these blocks become top level output ports or are discarded, depending on how they are configured."
  y_tbt_o7 : xbsIndex_r4/Gateway Out  inherit_from_input=on  hdl_port=off  timing_constraint=None  locs_specified=off  LOCs={}  UseAsDAC=off  DACChannel='1'  block_type=gatewayout
      settings: infoedit="Gateway out block.  Converts Xilinx fixed-point or floating-point type inputs into ouputs of type Simulink integer, single, double, or fixed point.<br><br>Hardware notes:  In hardware these blocks become top level output ports or are discarded, depending on how they are configured."
  wires:
  [Y_DIVIDEND_D_S_FPGA_RDY] -> q_tbt_o3/1
  [Y_DIVIDEND_D_S_FPGA] -> x_tbt_o3/1
  x_tbt_o3/1 -> D_S3/1
  [SUM_DIVISOR_D_S_FPGA] -> x_tbt_o4/1
  [SUM_DIVISOR_D_S_FPGA_VALID] -> y_tbt_o4/1
  x_tbt_o4/1 -> D_S3/3
  y_tbt_o4/1 -> D_S3/4
  [D_S_FPGA_Y_DIVIDER_QUOC] -> y_tbt_o7/1
  y_tbt_o7/1 -> D_S4/3
  Constant/1 -> D_S4/4
  q_tbt_o3/1 -> D_S2/1
  Constant1/1 -> D_S4/1
  Constant2/1 -> D_S4/2
  Constant3/1 -> D_S3/2
  [Y_DIVIDOR_D_S_FPGA_RDY] -> sum_tbt_o3/1
  sum_tbt_o3/1 -> D_S2/2
